simulink model "dma_fifo"  (R2020a)
settings: Solver=VariableStepAuto  StartTime=0.0  StopTime=10.0  RelTol=1e-3
libraries: hdlsllib x2
settings Model: Creator=sunip  LastModifiedBy=sunip
settings OptimizationCC: DefaultParameterBehavior=Inlined

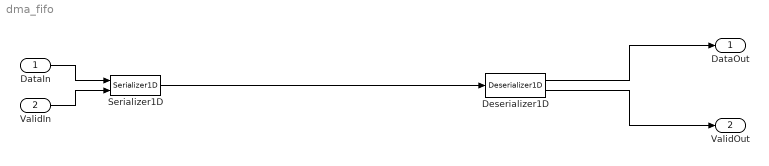
== system dma_fifo ==
  DataIn : Inport  OutDataTypeStr=uint32  SampleTime=0.001
  ValidIn : Inport  Port=2  OutDataTypeStr=boolean  SampleTime=0.001
  Deserializer1D : hdlsllib/HDL Operations/Deserializer1D  Ratio=1  IdleCycles=0  InitialCondition=0  startIn=off  validIn=off  validOut=on  inputDataDimensions=-1  inputSampleTime=-1  inputSignalType=auto
      settings: SourceProductBaseCode=SL
  Serializer1D : hdlsllib/HDL Operations/Serializer1D  Ratio=1  IdleCycles=0  validIn=on  startOut=off  validOut=off  inputDataDimensions=-1  inputSampleTime=-1  inputSignalType=auto
      settings: SourceProductBaseCode=SL
  DataOut : Outport  OutDataTypeStr=uint32
  ValidOut : Outport  Port=2  OutDataTypeStr=boolean
  wires:
  Deserializer1D/2 -> ValidOut/1
  DataIn/1 -> Serializer1D/1
  Deserializer1D/1 -> DataOut/1
  ValidIn/1 -> Serializer1D/2
  Serializer1D/1 -> Deserializer1D/1
